simulink model "tustinintegrator"  (R2021b)
settings: Solver=FixedStepDiscrete  StartTime=0.0  StopTime=10.0  FixedStep=0.1  RelTol=1e-3  EnableMultiTasking=on
model workspace (MAT data in the model file):
  BL = 8.23150537429
  F = [8.13150537429; 8.13142216591; 8.13133978892; 8.1312590664; 8.13118080491; 8.13110578641; 8.13103476046; 8.13096843672; 8.13090747789; 8.13085249304; 8.13080403157; 8.13076257768; 8.13072854557; 8.13070227528; 8.13068402928; 8.13067398989; 8.13067225743; 8.13067884918; 8.13069369931; 8.13071665942; 8.13074750011; 8.13078591323; 8.13083151497; 8.13088384969; 8.13094239447; 8.13100656436; 8.1310757182; 8.13114916502; 8.13122617096; 8.13130596661; 8.13138775468; 8.13147071796; 8.18987951772; 8.28925106843; 8.38704647632; 8.48228860198; 8.57402581759; 8.6613415152; 8.74336326523; 8.81927153347; 8.8883078696; 8.94978248536; 9.0030811467; 9.04767131104; 9.08310744818; 9.10903549196; 9.12519637792; 9.13142863185; 9.13142549913; 9.13141407056; 9.13139446034; 9.13136686441; 9.13133155851; 9.13128889538; 9.13123930132; 9.13118327185; 9.13112136679; 9.13105420468; 9.13098245659; 9.13090683939; 9.13082810863; 9.13074705096; 9.13066447627; 9.13058120964; 9.13049808303; 9.13041592702; 9.13033556248; 9.13025779239; 9.13018339379; 9.13011311007; 9.13004764346; 9.12998764809; 9.12993372342; 9.12988640823; 9.1298461753; 9.12981342661; 9.12978848937; 9.12977161276; 9.12976296539; 9.12976263367; 9.12977062091; 9.12978684731; 9.12981115074; 9.12984328837; 9.12988293908; 9.12992970671; 9.12998312396; 9.1300426571; 9.13010771131; 9.13017763658; 9.13025173424; 9.13032926393; 9.130409451; 9.13049149425; 9.13057457393; 9.13065785994; 9.1307405201; 9.1308217285; 9.13090067375; 9.13097656704; 9.13104865006]
  FR = [0; 0]
  Ft = 9.13104865006
  InputSize = 2
  M = [-0.839071529076 11.6908735095 8.23150537429 0 7.20521060927 8.68702753918 101 9.13104865006]
  N = 30
  NoXin = 11
  T = 0.1
  TL = 11.6908735095
  Tb = table
  Tb.data = {-0.839071529076, 11.6908735095, 8.23150537429, 0, 7.20521060927, 8.68702753918, 101, 9.13104865006}
  Tb.ndims = 2
  Tb.nrows = 1
  Tb.nvars = 8
  Tb.varnames = {'Var1', 'TL', 'BL', 'reset', 'ic', 'Var6', 'i', 'Ft'}
  Tb.props.useVariableNamesOriginal = 0
  Tb.props.useDimensionNamesOriginal = 0
  Tb.props.CustomProps = struct()
  Tb.props.VariableCustomProps = struct()
  Tb.props.versionSavedFrom = 4
  Tb.props.minCompatibleVersion = 1
  Tb.props.incompatibilityMsg = ''
  Tb.props.VersionSavedFrom = 4
  Tb.props.Description = ''
  Tb.props.VariableNamesOriginal = {}
  Tb.props.DimensionNames = {'Row', 'Variables'}
  Tb.props.DimensionNamesOriginal = {}
  Tb.props.UserData = []
  Tb.props.VariableDescriptions = {}
  Tb.props.VariableUnits = {}
  Tb.props.VariableContinuity = {}
  TimeSteps = 11
  Tt = table
  Tt.data = {-9.07788040727, -8.16497170243, 7.30766247044, -2.32776295076, 0, 1.42362489742, -2.32776295076, -2.32776295076, -3.18990555625, 0.8621}
  Tt.ndims = 2
  Tt.nrows = 1
  Tt.nvars = 10
  Tt.varnames = {'Var1', 'Var2', 'TL', 'BL', 'reset', 'ic', 'Var7', 'Var8', 'Var9', 'Ft'}
  Tt.props.useVariableNamesOriginal = 0
  Tt.props.useDimensionNamesOriginal = 0
  Tt.props.CustomProps = struct()
  Tt.props.VariableCustomProps = struct()
  Tt.props.versionSavedFrom = 4
  Tt.props.minCompatibleVersion = 1
  Tt.props.incompatibilityMsg = ''
  Tt.props.VersionSavedFrom = 4
  Tt.props.Description = ''
  Tt.props.VariableNamesOriginal = {}
  Tt.props.DimensionNames = {'Row', 'Variables'}
  Tt.props.DimensionNamesOriginal = {}
  Tt.props.UserData = []
  Tt.props.VariableDescriptions = {}
  Tt.props.VariableUnits = {}
  Tt.props.VariableContinuity = {}
  X = [-5.79809349406 -13.1040780606 -1.24495828784 -9.02552688812 -0.433163272214 -17.2538016032 -18.8945489592 -16.51912605 1.81655134952 18.7577752343 -0.666271750727 -8.10278974593 -4.40052552155 -19.0530783869]
  Xin = [-6.38459740191; -10.9336737451; -10.2920693381; 0.11665630484; 15.3990498967; -14.7573422555; -13.99000329; -10.0262082368; 12.5713930428; -6.46038302685; -12.2050634083]
  XmosomeSize = 15
  cs : handle (value not decoded)
  curPath = 'C:\Python-Workspace\thesis\FSE2019_latest\ModeTestingData\Problems'
  hws = Simulink.ModelWorkspace
  i = 6
  ic = 7.20521060927
  j = 6
  list(1).name = 'BL'
  list(1).size = [1 1]
  list(1).bytes = 8
  list(1).class = 'double'
  list(1).global = 0
  list(1).sparse = 0
  list(1).complex = 0
  list(1).nesting.function = 'simtstn'
  list(1).nesting.level = 1
  list(1).persistent = 0
  list(2).name = 'F'
  list(2).size = [101 1]
  list(2).bytes = 808
  list(2).class = 'double'
  list(2).global = 0
  list(2).sparse = 0
  list(2).complex = 0
  list(2).nesting.function = 'simtstn'
  list(2).nesting.level = 1
  list(2).persistent = 0
  list(3).name = 'FR'
  list(3).size = [2 1]
  list(3).bytes = 16
  list(3).class = 'double'
  list(3).global = 0
  list(3).sparse = 0
  list(3).complex = 0
  list(3).nesting.function = 'simtstn'
  list(3).nesting.level = 1
  list(3).persistent = 0
  list(4).name = 'Ft'
  list(4).size = [1 1]
  list(4).bytes = 8
  list(4).class = 'double'
  list(4).global = 0
  list(4).sparse = 0
  list(4).complex = 0
  list(4).nesting.function = 'simtstn'
  list(4).nesting.level = 1
  list(4).persistent = 0
  list(5).name = 'InputSize'
  list(5).size = [1 1]
  list(5).bytes = 8
  list(5).class = 'double'
  list(5).global = 0
  list(5).sparse = 0
  list(5).complex = 0
  list(5).nesting.function = 'simtstn'
  list(5).nesting.level = 1
  list(5).persistent = 0
  list(6).name = 'M'
  list(6).size = [1 8]
  list(6).bytes = 64
  list(6).class = 'double'
  list(6).global = 0
  list(6).sparse = 0
  list(6).complex = 0
  list(6).nesting.function = 'simtstn'
  list(6).nesting.level = 1
  list(6).persistent = 0
  list(7).name = 'N'
  list(7).size = [1 1]
  list(7).bytes = 8
  list(7).class = 'double'
  list(7).global = 0
  list(7).sparse = 0
  list(7).complex = 0
  list(7).nesting.function = 'simtstn'
  list(7).nesting.level = 1
  list(7).persistent = 0
  list(8).name = 'T'
  list(8).size = [1 1]
  list(8).bytes = 8
  list(8).class = 'double'
  list(8).global = 0
  list(8).sparse = 0
  list(8).complex = 0
  list(8).nesting.function = 'simtstn'
  list(8).nesting.level = 1
  list(8).persistent = 0
  list(9).name = 'TL'
  list(9).size = [1 1]
  list(9).bytes = 8
  list(9).class = 'double'
  list(9).global = 0
  list(9).sparse = 0
  list(9).complex = 0
  list(9).nesting.function = 'simtstn'
  list(9).nesting.level = 1
  list(9).persistent = 0
  list(10).name = 'Tb'
  list(10).size = [1 8]
  list(10).bytes = 3154
  list(10).class = 'table'
  list(10).global = 0
  list(10).sparse = 0
  list(10).complex = 0
  list(10).nesting.function = 'simtstn'
  list(10).nesting.level = 1
  list(10).persistent = 0
  list(11).name = 'TimeSteps'
  list(11).size = [1 1]
  list(11).bytes = 8
  list(11).class = 'double'
  list(11).global = 0
  list(11).sparse = 0
  list(11).complex = 0
  list(11).nesting.function = 'simtstn'
  list(11).nesting.level = 1
  list(11).persistent = 0
  list(12).name = 'X'
  list(12).size = [2 3]
  list(12).bytes = 48
  list(12).class = 'double'
  list(12).global = 0
  list(12).sparse = 0
  list(12).complex = 0
  list(12).nesting.function = 'simtstn'
  list(12).nesting.level = 1
  list(12).persistent = 0
  list(13).name = 'cs'
  list(13).size = [1 1]
  list(13).bytes = 0
  list(13).class = 'Simulink.ConfigSet'
  list(13).global = 0
  list(13).sparse = 0
  list(13).complex = 0
  list(13).nesting.function = 'simtstn'
  list(13).nesting.level = 1
  list(13).persistent = 0
  list(14).name = 'curPath'
  list(14).size = [1 81]
  list(14).bytes = 162
  list(14).class = 'char'
  list(14).global = 0
  list(14).sparse = 0
  list(14).complex = 0
  list(14).nesting.function = 'simtstn'
  list(14).nesting.level = 1
  list(14).persistent = 0
  list(15).name = 'hws'
  list(15).size = [1 1]
  list(15).bytes = 0
  list(15).class = 'Simulink.ModelWorkspace'
  list(15).global = 0
  list(15).sparse = 0
  list(15).complex = 0
  list(15).nesting.function = 'simtstn'
  list(15).nesting.level = 1
  list(15).persistent = 0
  list(16).name = 'i'
  list(16).size = [1 1]
  list(16).bytes = 8
  list(16).class = 'double'
  list(16).global = 0
  list(16).sparse = 0
  list(16).complex = 0
  list(16).nesting.function = 'simtstn'
  list(16).nesting.level = 1
  list(16).persistent = 0
  list(17).name = 'ic'
  list(17).size = [1 1]
  list(17).bytes = 8
  list(17).class = 'double'
  list(17).global = 0
  list(17).sparse = 0
  list(17).complex = 0
  list(17).nesting.function = 'simtstn'
  list(17).nesting.level = 1
  list(17).persistent = 0
  list(18).name = 'j'
  list(18).size = [1 1]
  list(18).bytes = 8
  list(18).class = 'double'
  list(18).global = 0
  list(18).sparse = 0
  list(18).complex = 0
  list(18).nesting.function = 'simtstn'
  list(18).nesting.level = 1
  list(18).persistent = 0
  list(19).name = 'list'
  list(19).size = [14 1]
  list(19).bytes = 20688
  list(19).class = 'struct'
  list(19).global = 0
  list(19).sparse = 0
  list(19).complex = 0
  list(19).nesting.function = 'simtstn'
  list(19).nesting.level = 1
  list(19).persistent = 0
  list(20).name = 'model_cs'
  list(20).size = [1 1]
  list(20).bytes = 0
  list(20).class = 'Simulink.ConfigSet'
  list(20).global = 0
  list(20).sparse = 0
  list(20).complex = 0
  list(20).nesting.function = 'simtstn'
  list(20).nesting.level = 1
  list(20).persistent = 0
  list(21).name = 'modelpath'
  list(21).size = [1 81]
  list(21).bytes = 162
  list(21).class = 'char'
  list(21).global = 0
  list(21).sparse = 0
  list(21).complex = 0
  list(21).nesting.function = 'simtstn'
  list(21).nesting.level = 1
  list(21).persistent = 0
  list(22).name = 'n'
  list(22).size = [1 1]
  list(22).bytes = 8
  list(22).class = 'double'
  list(22).global = 0
  list(22).sparse = 0
  list(22).complex = 0
  list(22).nesting.function = 'simtstn'
  list(22).nesting.level = 1
  list(22).persistent = 0
  list(23).name = 'nbrInputs'
  list(23).size = [1 1]
  list(23).bytes = 8
  list(23).class = 'double'
  list(23).global = 0
  list(23).sparse = 0
  list(23).complex = 0
  list(23).nesting.function = 'simtstn'
  list(23).nesting.level = 1
  list(23).persistent = 0
  list(24).name = 'reset'
  list(24).size = [1 1]
  list(24).bytes = 8
  list(24).class = 'double'
  list(24).global = 0
  list(24).sparse = 0
  list(24).complex = 0
  list(24).nesting.function = 'simtstn'
  list(24).nesting.level = 1
  list(24).persistent = 0
  list(25).name = 'simOut'
  list(25).size = [1 1]
  list(25).bytes = 10012
  list(25).class = 'Simulink.SimulationOutput'
  list(25).global = 0
  list(25).sparse = 0
  list(25).complex = 0
  list(25).nesting.function = 'simtstn'
  list(25).nesting.level = 1
  list(25).persistent = 0
  list(26).name = 't'
  list(26).size = [101 1]
  list(26).bytes = 808
  list(26).class = 'double'
  list(26).global = 0
  list(26).sparse = 0
  list(26).complex = 0
  list(26).nesting.function = 'simtstn'
  list(26).nesting.level = 1
  list(26).persistent = 0
  list(27).name = 'var'
  list(27).size = [1 1]
  list(27).bytes = 7528
  list(27).class = 'struct'
  list(27).global = 0
  list(27).sparse = 0
  list(27).complex = 0
  list(27).nesting.function = 'simtstn'
  list(27).nesting.level = 1
  list(27).persistent = 0
  list(28).name = 'varout'
  list(28).size = [1 1]
  list(28).bytes = 2722
  list(28).class = 'struct'
  list(28).global = 0
  list(28).sparse = 0
  list(28).complex = 0
  list(28).nesting.function = 'simtstn'
  list(28).nesting.level = 1
  list(28).persistent = 0
  list(29).name = 'xin'
  list(29).size = [101 1]
  list(29).bytes = 808
  list(29).class = 'double'
  list(29).global = 0
  list(29).sparse = 0
  list(29).complex = 0
  list(29).nesting.function = 'simtstn'
  list(29).nesting.level = 1
  list(29).persistent = 0
  list(30).name = 'y'
  list(30).size = [101 1]
  list(30).bytes = 808
  list(30).class = 'double'
  list(30).global = 0
  list(30).sparse = 0
  list(30).complex = 0
  list(30).nesting.function = 'simtstn'
  list(30).nesting.level = 1
  list(30).persistent = 0
  model_cs : handle (value not decoded)
  modelpath = 'C:\Python-Workspace\thesis\FSE2019_latest\Benchmark\Simulink Models\2_tustin\'
  n = 1
  nbrInputs = 6
  req = 'R1c'
  reset = 0
  s = 6
  simOut = Simulink.SimulationOutput
  simOut.Data.tout = [0; 0.1; 0.2; 0.3; 0.4; 0.5; 0.6; 0.7; 0.8; 0.9; 1; 1.1; 1.2; 1.3; 1.4; 1.5; 1.6; 1.7; 1.8; 1.9; 2; 2.1; 2.2; 2.3; 2.4; 2.5; 2.6; 2.7; 2.8; 2.9; 3; 3.1; 3.2; 3.3; 3.4; 3.5; 3.6; 3.7; 3.8; 3.9; 4; 4.1; 4.2; 4.3; 4.4; 4.5; 4.6; 4.7; 4.8; 4.9; 5; 5.1; 5.2; 5.3; 5.4; 5.5; 5.6; 5.7; 5.8; 5.9; 6; 6.1; 6.2; 6.3; 6.4; 6.5; 6.6; 6.7; 6.8; 6.9; 7; 7.1; 7.2; 7.3; 7.4; 7.5; 7.6; 7.7; 7.8; 7.9; 8; 8.1; 8.2; 8.3; 8.4; 8.5; 8.6; 8.7; 8.8; 8.9; 9; 9.1; 9.2; 9.3; 9.4; 9.5; 9.6; 9.7; 9.8; 9.9; 10]
  simOut.Data.varout.time = [0; 0.1; 0.2; 0.3; 0.4; 0.5; 0.6; 0.7; 0.8; 0.9; 1; 1.1; 1.2; 1.3; 1.4; 1.5; 1.6; 1.7; 1.8; 1.9; 2; 2.1; 2.2; 2.3; 2.4; 2.5; 2.6; 2.7; 2.8; 2.9; 3; 3.1; 3.2; 3.3; 3.4; 3.5; 3.6; 3.7; 3.8; 3.9; 4; 4.1; 4.2; 4.3; 4.4; 4.5; 4.6; 4.7; 4.8; 4.9; 5; 5.1; 5.2; 5.3; 5.4; 5.5; 5.6; 5.7; 5.8; 5.9; 6; 6.1; 6.2; 6.3; 6.4; 6.5; 6.6; 6.7; 6.8; 6.9; 7; 7.1; 7.2; 7.3; 7.4; 7.5; 7.6; 7.7; 7.8; 7.9; 8; 8.1; 8.2; 8.3; 8.4; 8.5; 8.6; 8.7; 8.8; 8.9; 9; 9.1; 9.2; 9.3; 9.4; 9.5; 9.6; 9.7; 9.8; 9.9; 10]
  simOut.Data.varout.signals.values = [8.23150537429; 8.33125558255; 8.43000911971; 8.52677927306; 8.62059914722; 8.71053132501; 8.79567723385; 8.87518612396; 8.94826356879; 9.01417940267; 9.07227501638; 9.12196993774; 9.16276763154; 9.19426046069; 9.21613375927; 9.2281689765; 9.23024586047; 9.22234365964; 9.20454133019; 9.17701674711; 9.14004492694; 9.09399527988; 9.03932791879; 8.97658906186; 8.90640557502; 8.82947870847; 8.74657709002; 8.65852904525; 8.56621432112; 8.47055529583; 8.37250776274; 8.2730513804; 8.23150537429; 8.23150537429; 8.23150537429; 8.23150537429; 8.23150537429; 8.23150537429; 8.23150537429; 8.23150537429; 8.23150537429; 8.23150537429; 8.23150537429; 8.23150537429; 8.23150537429; 8.23150537429; 8.23150537429; 8.23150537429; 8.23526089029; 8.24896145793; 8.27247018568; 8.30555218209; 8.34787690279; 8.39902145316; 8.45847481377; 8.52564294628; 8.59985472892; 8.68036866209; 8.76638027717; 8.85703017456; 8.95141261043; 9.04858454668; 9.14757507346; 9.24739511013; 9.34704728788; 9.44553591511; 9.54187692599; 9.635107713; 9.72429674493; 9.80855287446; 9.88703424218; 9.95895668822; 10.0236015873; 10.0803230289; 10.1285542711; 10.1678134034; 10.1977081614; 10.2179398466; 10.2283063108; 10.2287039755; 10.2191288675; 10.1996766582; 10.1705417074; 10.1320151221; 10.0844818472; 10.0284168193; 9.96438022183; 9.89301188719; 9.8150249042; 9.73119849304; 9.64237021948; 9.54942762628; 9.4532993651; 9.35494591776; 9.25534999939; 9.15550673947; 9.05641373887; 8.95906110209; 8.8644215445; 8.77344067326; 8.68702753918]
  simOut.Data.varout.signals.dimensions = 1
  simOut.Data.varout.signals.label = ''
  simOut.Data.varout.signals.blockName = 'tustinintegrator/yout'
  simOut.Metadata = Simulink.SimulationMetadata
  simOut.Metadata.ModelInfo.ModelName = 'tustinintegrator'
  simOut.Metadata.ModelInfo.ModelVersion = '1.55'
  simOut.Metadata.ModelInfo.ModelFilePath = '/Users/ceren.gebizli/Desktop/Shiva/QRA-Search/QRA-Search/SimulinkModels/2_tustin/tustinintegrator.slx'
  simOut.Metadata.ModelInfo.UserID = 'ceren.gebizli'
  simOut.Metadata.ModelInfo.MachineName = ''
  simOut.Metadata.ModelInfo.Platform = 'MACI64'
  simOut.Metadata.ModelInfo.ModelStructuralChecksum = [3314600462; 258222661; 2212550858; 2950727440]
  simOut.Metadata.ModelInfo.SimulationMode = 'normal'
  simOut.Metadata.ModelInfo.StartTime = 0
  simOut.Metadata.ModelInfo.StopTime = 10
  simOut.Metadata.ModelInfo.SolverInfo.Type = 'Fixed-Step'
  simOut.Metadata.ModelInfo.SolverInfo.Solver = 'FixedStepDiscrete'
  simOut.Metadata.ModelInfo.SolverInfo.FixedStepSize = 0.1
  simOut.Metadata.ModelInfo.SimulinkVersion.Name = 'Simulink'
  simOut.Metadata.ModelInfo.SimulinkVersion.Version = '8.7'
  simOut.Metadata.ModelInfo.SimulinkVersion.Release = '(R2016a)'
  simOut.Metadata.ModelInfo.SimulinkVersion.Date = '10-Feb-2016'
  simOut.Metadata.TimingInfo.WallClockTimestampStart = '2018-06-06 16:28:47.251939'
  simOut.Metadata.TimingInfo.WallClockTimestampStop = '2018-06-06 16:28:47.966952'
  simOut.Metadata.TimingInfo.InitializationElapsedWallTime = 0.692111
  simOut.Metadata.TimingInfo.ExecutionElapsedWallTime = 0.000638
  simOut.Metadata.TimingInfo.TerminationElapsedWallTime = 0.022275
  simOut.Metadata.TimingInfo.TotalElapsedWallTime = 0.715024
  simOut.Metadata.ExecutionInfo.StopEvent = 'ReachedStopTime'
  simOut.Metadata.ExecutionInfo.StopEventSource = []
  simOut.Metadata.ExecutionInfo.StopEventDescription = 'Reached stop time of 10'
  simOut.Metadata.ExecutionInfo.ErrorDiagnostic = []
  simOut.Metadata.ExecutionInfo.WarningDiagnostics = struct([])
  simOut.Metadata.AppInfo = struct()
  t = [0; 0.1; 0.2; 0.3; 0.4; 0.5; 0.6; 0.7; 0.8; 0.9; 1; 1.1; 1.2; 1.3; 1.4; 1.5; 1.6; 1.7; 1.8; 1.9; 2; 2.1; 2.2; 2.3; 2.4; 2.5; 2.6; 2.7; 2.8; 2.9; 3; 3.1; 3.2; 3.3; 3.4; 3.5; 3.6; 3.7; 3.8; 3.9; 4; 4.1; 4.2; 4.3; 4.4; 4.5; 4.6; 4.7; 4.8; 4.9; 5; 5.1; 5.2; 5.3; 5.4; 5.5; 5.6; 5.7; 5.8; 5.9; 6; 6.1; 6.2; 6.3; 6.4; 6.5; 6.6; 6.7; 6.8; 6.9; 7; 7.1; 7.2; 7.3; 7.4; 7.5; 7.6; 7.7; 7.8; 7.9; 8; 8.1; 8.2; 8.3; 8.4; 8.5; 8.6; 8.7; 8.8; 8.9; 9; 9.1; 9.2; 9.3; 9.4; 9.5; 9.6; 9.7; 9.8; 9.9; 10]
  var.time = [0 1 2 3 4 5 6 7 8 9 10]
  var.signals(1).values = [-5.79809349406; -13.1040780606; -1.24495828784; -9.02552688812; -0.433163272214; -17.2538016032; -18.8945489592; -16.51912605; 1.81655134952; 18.7577752343; -0.666271750727]
  var.signals(1).dimensions = 1
  var.signals(2).values = [1; 1; 1; 1; 1; 1; 1; 1; 1; 1; 1]
  var.signals(2).dimensions = 1
  var.signals(3).values = [1; 1; 1; 1; 1; 1; 1; 1; 1; 1; 1]
  var.signals(3).dimensions = 1
  var.signals(4).values = [-19.0530783869; -19.0530783869; -19.0530783869; -19.0530783869; -19.0530783869; -19.0530783869; -19.0530783869; -19.0530783869; -19.0530783869; -19.0530783869; -19.0530783869]
  var.signals(4).dimensions = 1
  var.signals(5).values = [-8.10278974593; -8.10278974593; -8.10278974593; -8.10278974593; -8.10278974593; -8.10278974593; -8.10278974593; -8.10278974593; -8.10278974593; -8.10278974593; -8.10278974593]
  var.signals(5).dimensions = 1
  var.signals(6).values = [-4.40052552155; -4.40052552155; -4.40052552155; -4.40052552155; -4.40052552155; -4.40052552155; -4.40052552155; -4.40052552155; -4.40052552155; -4.40052552155; -4.40052552155]
  var.signals(6).dimensions = 1
  varout.time = [0; 0.1; 0.2; 0.3; 0.4; 0.5; 0.6; 0.7; 0.8; 0.9; 1; 1.1; 1.2; 1.3; 1.4; 1.5; 1.6; 1.7; 1.8; 1.9; 2; 2.1; 2.2; 2.3; 2.4; 2.5; 2.6; 2.7; 2.8; 2.9; 3; 3.1; 3.2; 3.3; 3.4; 3.5; 3.6; 3.7; 3.8; 3.9; 4; 4.1; 4.2; 4.3; 4.4; 4.5; 4.6; 4.7; 4.8; 4.9; 5; 5.1; 5.2; 5.3; 5.4; 5.5; 5.6; 5.7; 5.8; 5.9; 6; 6.1; 6.2; 6.3; 6.4; 6.5; 6.6; 6.7; 6.8; 6.9; 7; 7.1; 7.2; 7.3; 7.4; 7.5; 7.6; 7.7; 7.8; 7.9; 8; 8.1; 8.2; 8.3; 8.4; 8.5; 8.6; 8.7; 8.8; 8.9; 9; 9.1; 9.2; 9.3; 9.4; 9.5; 9.6; 9.7; 9.8; 9.9; 10]
  varout.signals.values = [8.23150537429; 8.33125558255; 8.43000911971; 8.52677927306; 8.62059914722; 8.71053132501; 8.79567723385; 8.87518612396; 8.94826356879; 9.01417940267; 9.07227501638; 9.12196993774; 9.16276763154; 9.19426046069; 9.21613375927; 9.2281689765; 9.23024586047; 9.22234365964; 9.20454133019; 9.17701674711; 9.14004492694; 9.09399527988; 9.03932791879; 8.97658906186; 8.90640557502; 8.82947870847; 8.74657709002; 8.65852904525; 8.56621432112; 8.47055529583; 8.37250776274; 8.2730513804; 8.23150537429; 8.23150537429; 8.23150537429; 8.23150537429; 8.23150537429; 8.23150537429; 8.23150537429; 8.23150537429; 8.23150537429; 8.23150537429; 8.23150537429; 8.23150537429; 8.23150537429; 8.23150537429; 8.23150537429; 8.23150537429; 8.23526089029; 8.24896145793; 8.27247018568; 8.30555218209; 8.34787690279; 8.39902145316; 8.45847481377; 8.52564294628; 8.59985472892; 8.68036866209; 8.76638027717; 8.85703017456; 8.95141261043; 9.04858454668; 9.14757507346; 9.24739511013; 9.34704728788; 9.44553591511; 9.54187692599; 9.635107713; 9.72429674493; 9.80855287446; 9.88703424218; 9.95895668822; 10.0236015873; 10.0803230289; 10.1285542711; 10.1678134034; 10.1977081614; 10.2179398466; 10.2283063108; 10.2287039755; 10.2191288675; 10.1996766582; 10.1705417074; 10.1320151221; 10.0844818472; 10.0284168193; 9.96438022183; 9.89301188719; 9.8150249042; 9.73119849304; 9.64237021948; 9.54942762628; 9.4532993651; 9.35494591776; 9.25534999939; 9.15550673947; 9.05641373887; 8.95906110209; 8.8644215445; 8.77344067326; 8.68702753918]
  varout.signals.dimensions = 1
  varout.signals.label = ''
  varout.signals.blockName = 'tustinintegrator/yout'
  xin = [1; 0.995004165278; 0.980066577841; 0.955336489126; 0.921060994003; 0.87758256189; 0.82533561491; 0.764842187284; 0.696706709347; 0.621609968271; 0.540302305868; 0.453596121426; 0.362357754477; 0.267498828625; 0.1699671429; 0.0707372016677; -0.0291995223013; -0.128844494296; -0.227202094693; -0.323289566864; -0.416146836547; -0.5048461046; -0.588501117255; -0.66627602128; -0.737393715541; -0.801143615547; -0.856888753369; -0.904072142017; -0.942222340669; -0.97095816515; -0.9899924966; -0.999135150273; -0.998294775795; -0.987479769909; -0.966798192579; -0.936456687291; -0.896758416334; -0.84810003171; -0.790967711914; -0.7259323042; -0.653643620864; -0.574823946533; -0.490260821341; -0.40079917208; -0.307332869978; -0.210795799431; -0.112152526935; -0.0123886634629; 0.0874989834394; 0.186512369423; 0.283662185463; 0.377977742713; 0.4685166713; 0.554374336179; 0.634692875943; 0.708669774291; 0.77556587851; 0.834712784839; 0.885519516941; 0.927478430744; 0.96017028665; 0.983268438443; 0.996542097023; 0.999858636383; 0.993184918758; 0.976587625728; 0.950232591959; 0.914383148235; 0.86939749035; 0.815725100125; 0.753902254343; 0.684546666443; 0.608351314532; 0.526077517381; 0.438547327574; 0.346635317835; 0.251259842582; 0.153373862038; 0.0539554205626; -0.0460021256395; -0.145500033809; -0.243544153736; -0.339154860984; -0.431376844971; -0.519288654117; -0.602011902685; -0.67872004732; -0.748646645597; -0.811093014062; -0.865435209241; -0.911130261885; -0.947721602131; -0.974843621404; -0.992225325453; -0.999693042035; -0.997172156196; -0.984687855794; -0.962364879831; -0.930426272105; -0.889191152625; -0.839071529076]
  y = [8.23150537429; 8.33125558255; 8.43000911971; 8.52677927306; 8.62059914722; 8.71053132501; 8.79567723385; 8.87518612396; 8.94826356879; 9.01417940267; 9.07227501638; 9.12196993774; 9.16276763154; 9.19426046069; 9.21613375927; 9.2281689765; 9.23024586047; 9.22234365964; 9.20454133019; 9.17701674711; 9.14004492694; 9.09399527988; 9.03932791879; 8.97658906186; 8.90640557502; 8.82947870847; 8.74657709002; 8.65852904525; 8.56621432112; 8.47055529583; 8.37250776274; 8.2730513804; 8.23150537429; 8.23150537429; 8.23150537429; 8.23150537429; 8.23150537429; 8.23150537429; 8.23150537429; 8.23150537429; 8.23150537429; 8.23150537429; 8.23150537429; 8.23150537429; 8.23150537429; 8.23150537429; 8.23150537429; 8.23150537429; 8.23526089029; 8.24896145793; 8.27247018568; 8.30555218209; 8.34787690279; 8.39902145316; 8.45847481377; 8.52564294628; 8.59985472892; 8.68036866209; 8.76638027717; 8.85703017456; 8.95141261043; 9.04858454668; 9.14757507346; 9.24739511013; 9.34704728788; 9.44553591511; 9.54187692599; 9.635107713; 9.72429674493; 9.80855287446; 9.88703424218; 9.95895668822; 10.0236015873; 10.0803230289; 10.1285542711; 10.1678134034; 10.1977081614; 10.2179398466; 10.2283063108; 10.2287039755; 10.2191288675; 10.1996766582; 10.1705417074; 10.1320151221; 10.0844818472; 10.0284168193; 9.96438022183; 9.89301188719; 9.8150249042; 9.73119849304; 9.64237021948; 9.54942762628; 9.4532993651; 9.35494591776; 9.25534999939; 9.15550673947; 9.05641373887; 8.95906110209; 8.8644215445; 8.77344067326; 8.68702753918]
  ycomp = [0.180453367991; 0.642647312322; 1.80047084027; 2.95440128824; 3.94847654161; 5.09308941904; 5.25147536168; 5.35667142697; 6.68987387998; 7.32044632308; 7.97311703367; 8.56340422856; 8.20631949486; 6.96915318731; 6.02137556346; 5.400585167; 5.4106738168; 7.04487036937; 8.19471931131; 6.64110253577; 5.16316495878; 4.56562739642; 4.90290282798; 4.38996762486; 2.87813907167; 1.97248289274; 1.84731469613; 1.2908620764; 0.226392499249; -0.0822196239338; 0.871876822815; 1.31870977116; 0.443383389599; 0.575058233531; 1.27343914636; 0.551208545524; 0.0409308967751; -0.466335286697; -0.617503069427; -0.00902839372751; 0.771157952585; 2.01128256287; 1.59240863428; 0.724305743189; 0.876831391533; 1.27618892046; 1.29432210905; 1.84815762198; 1.78028355032; 1.78530408348; 1.83276335995; 0.202612424309; -0.220504577106; 0.475974540576; 0.996876080914; 1.09001719365; 0.125207539406; -0.408406848821; 0.0690776511744; 0.454881367133; 1.03127182553; 0.895293582777; -0.295862595662; -1.44523701318; -1.68130451404; -1.90379423209; -2.58129606919; -3.15349662446; -2.75622615746; -2.61772402031; -2.010376568; -1.31331238974; -2.02151132828; -1.90621006585; -2.13009388187; -3.46052410983; -2.06584760502; -2.35447994077; -3.33531972738; -3.31420254158; -3.09128137519; -2.30337688676; -2.84029338264; -3.18990555625; -1.78986153935; 0.0663726017768; -0.00642792921309; -0.428276000968; -0.348584612224; -0.437686126439; 0.809761537848; 1.50045115751; 0.652620282861; -0.50739756993; -0.132310340102; 1.64786061638; 1.59463704179; 0.246327580193; 0.563004598668; 0.431525551081; -0.982322159793]
libraries: simulink x1
settings Model: Creator=elliocm  LastModifiedBy=achan260
settings SolverCC: AlgebraicLoopSolver=TrustRegion
settings DataIOCC: ExternalInput=var  LimitDataPoints=on  LoadExternalInput=on  SaveFormat=StructureWithTime  ReturnWorkspaceOutputs=off  OutputSaveName=varout
settings OptimizationCC: ExpressionDepthLimit=2147483647  LifeSpan=inf
settings DebuggingCC: UnderspecifiedInitializationDetection=Classic  MergeDetectMultiDrivingBlocksExec=none  SolverPrmCheckMsg=warning  IntegerOverflowMsg=none  StateNameClashWarn=warning  SFUnexpectedBacktrackingDiag=warning  SFNoUnconditionalDefaultTransitionDiag=warning  SFMachineParentedDataDiag=warning  IntegerSaturationMsg=none  ArithmeticOperatorsInVariantConditions=warning
settings HardwareCC: ProdBitPerPointer=32  ProdBitPerSizeT=32  ProdBitPerPtrDiffT=32  ProdLargestAtomicFloat=None  ProdIntDivRoundTo=Undefined  ProdEndianess=Unspecified  ProdWordSize=32  ProdHWDeviceType=32-bit Generic
settings ModelReferenceCC: PropagateSignalLabelsOutOfModel=off
settings SFSimCC: SimUseLocalCustomCode=off  CustomCodeUndefinedFunction=UseInterfaceOnly
settings RTWCC: RTWUseLocalCustomCode=off
settings CodeAppCC: StateflowObjectComments=on
settings GRTTargetCC: TargetLangStandard=C89/C90 (ANSI)
settings ConfigComp: CovMetricSettings=dw  CovSaveCumulativeToWorkspaceVar=on  CovSaveSingleToWorkspaceVar=on  CovExternalEMLEnable=off  DVMaxProcessTime=5000  DVMaxTestCaseSteps=500  DVTestSuiteOptimization=CombinedObjectives (Nonlinear Extended)  DVDetectActiveLogic=on

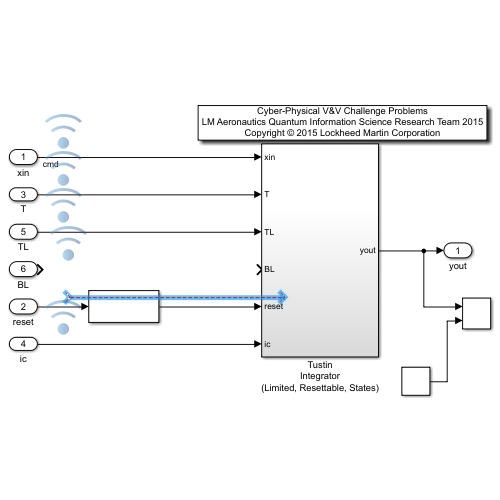
[thumbnail: Simulink's stored preview of the top-level diagram]
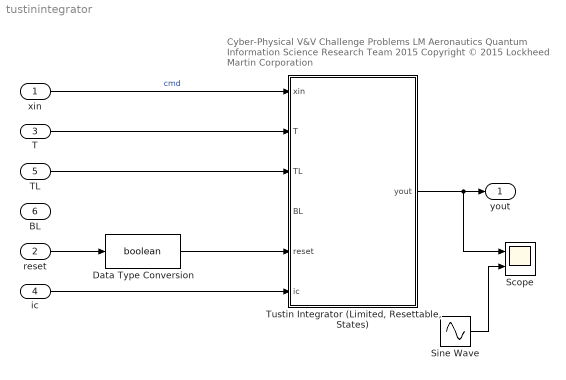
== system tustinintegrator ==
  note: Cyber-Physical V&V Challenge Problems
      | LM Aeronautics Quantum Information Science Research Team 2015
      | Copyright © 2015 Lockheed Martin Corporation
  xin : Inport  OutDataTypeStr=double  PortDimensions=1
  reset : Inport  Port=2  OutDataTypeStr=double
  T : Inport  Port=3  OutDataTypeStr=double
  ic : Inport  Port=4  OutDataTypeStr=double
  TL : Inport  Port=5  OutDataTypeStr=double
  BL : Inport  Port=6  OutDataTypeStr=double
  Data Type Conversion : DataTypeConversion  OutDataTypeStr=boolean
  Scope : Scope  NumInputPorts=2
  Sine Wave : Sin  SampleTime=0
  "Tustin Integrator (Limited, Resettable, States)" : Subsystem
  yout : Outport
  wires:
  TL/1 -> "Tustin Integrator (Limited, Resettable, States)"/3(TL)
  ic/1 -> "Tustin Integrator (Limited, Resettable, States)"/6(ic)
  "Tustin Integrator (Limited, Resettable, States)"/1(yout) -> Scope/1, yout/1
  T/1 -> "Tustin Integrator (Limited, Resettable, States)"/2(T)
  xin/1 -> "Tustin Integrator (Limited, Resettable, States)"/1(xin)  "cmd"
  reset/1 -> Data Type Conversion/1
  Data Type Conversion/1 -> "Tustin Integrator (Limited, Resettable, States)"/5(reset)
  Sine Wave/1 -> Scope/2
  ? -> ?

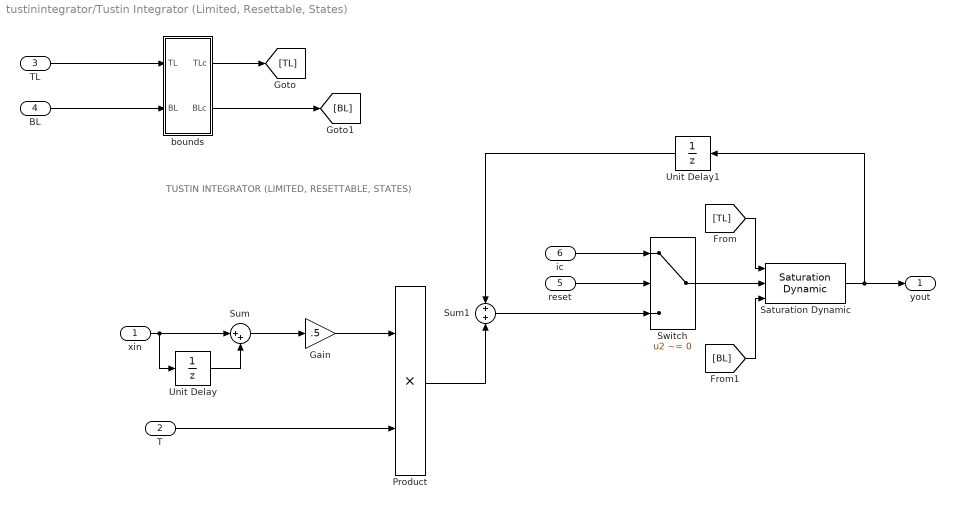
== system tustinintegrator/Tustin Integrator (Limited, Resettable, States) ==
  note: TUSTIN INTEGRATOR (LIMITED, RESETTABLE, STATES)
  xin : Inport
  T : Inport  Port=2
  TL : Inport  Port=3
  BL : Inport  Port=4
  reset : Inport  Port=5
  ic : Inport  Port=6
  Gain : Gain  Gain=.5
  Product : Product  RndMeth=Zero
  Saturation Dynamic : simulink/Discontinuities/Saturation Dynamic  OutMin=[]  OutMax=[]  OutDataTypeStr=Inherit: Same as second input  OutDataType=fixdt(1, 16)  OutScaling=2^-10  DoSatur=off
  Sum : Sum  Inputs=|++
  Sum1 : Sum
  Switch : Switch  Criteria=u2 ~= 0  Threshold=0.5
  Unit Delay : UnitDelay  SampleTime=-1  HasFrameUpgradeWarning=on
  Unit Delay1 : UnitDelay  SampleTime=-1  HasFrameUpgradeWarning=on
  bounds : Subsystem
  yout : Outport
  wires:
  xin/1 -> Unit Delay/1, Sum/1
  Unit Delay/1 -> Sum/2
  Sum/1 -> Gain/1
  Gain/1 -> Product/1
  T/1 -> Product/2
  Product/1 -> Sum1/2
  Sum1/1 -> Switch/3
  reset/1 -> Switch/2
  ic/1 -> Switch/1
  Switch/1 -> Saturation Dynamic/2
  Saturation Dynamic/1 -> Unit Delay1/1, yout/1
  Unit Delay1/1 -> Sum1/1
  TL/1 -> bounds/1(TL)
  BL/1 -> bounds/2(BL)
  bounds/1(TLc) -> [TL]
  bounds/2(BLc) -> [BL]
  [TL] -> Saturation Dynamic/1
  [BL] -> Saturation Dynamic/3

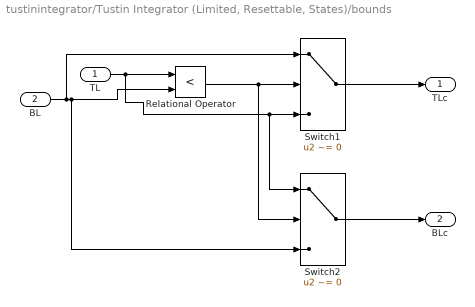
== system tustinintegrator/Tustin Integrator (Limited, Resettable, States)/bounds ==
  TL : Inport
  BL : Inport  Port=2
  Relational Operator : RelationalOperator  Operator=<  OutDataTypeStr=boolean  RndMeth=Nearest
  Switch1 : Switch  Criteria=u2 ~= 0  Threshold=0.5
  Switch2 : Switch  Criteria=u2 ~= 0  Threshold=0.5
  TLc : Outport
  BLc : Outport  Port=2
  wires:
  BL/1 -> Switch1/1, Switch2/3, Relational Operator/2
  TL/1 -> Switch2/1, Switch1/3, Relational Operator/1
  Relational Operator/1 -> Switch2/2, Switch1/2
  Switch1/1 -> TLc/1
  Switch2/1 -> BLc/1
